simulink model "mg_simulator"  (Simulink 9.0)
settings: Solver=VariableStepAuto  StartTime=0.0  StopTime=Tsim  FixedStep=.005  MaxStep=Ts  RelTol=1e-6  EnableMultiTasking=on
InitFcn:
  | mg_simulator_init
values from neighbouring files (symbols this model uses):
  g_vector = [1 1 1 1]    [mg_simulator_init.m]
  Init = [305; 297; 315; 320]    [mg_simulator_init.m]
  N = 3    [mg_simulator_init.m]    (also in mpc_run_nodewise2.m = 6; mpc_run_nodewise3.m = 6; mpc_run_nodewise4.m = 6; mpc_run_nodewise_slow.m = 6)
  n_Q1 = .01    (= 0.01)    [mg_simulator_init.m]
  n_Q2 = n_Q1    (= 0.01)    [mg_simulator_init.m]
  n_Q3 = n_Q2    (= 0.01)    [mg_simulator_init.m]
  n_Q4 = n_Q3    (= 0.01)    [mg_simulator_init.m]
  Q = 10*eye    [mg_simulator_init.m]    (also in mpc_run_nodewise2.m; mpc_run_nodewise3.m; mpc_run_nodewise4.m; mpc_run_nodewise_slow.m)
  R = .1*eye    [mg_simulator_init.m]    (also in mpc_run_nodewise2.m = 0*eye; mpc_run_nodewise3.m = 0*eye; mpc_run_nodewise4.m = 0*eye; mpc_run_nodewise_slow.m = 0*eye)
  Thresh = 4    [mg_simulator_init.m]
  Ts = .01    (= 0.01)    [mg_simulator_init.m]    (also in mpc_run_nodewise2.m = 0.3; mpc_run_nodewise3.m = 0.3; mpc_run_nodewise4.m = 0.3; mpc_run_nodewise_slow.m = 0.3)
  v_ref = 310    [mg_simulator_init.m]    (also in mpc_run_nodewise2.m; mpc_run_nodewise3.m; mpc_run_nodewise4.m; mpc_run_nodewise_slow.m)
undefined symbols (not defined in the file or in its folder): mpc_run_nodewise_mdl_fast, mpc_run_nodewise_mdl_fast2, mpc_run_nodewise_mdl_fast3, mpc_run_nodewise_mdl_fast4, plecs
settings Model: SuppressorTable=22 serialization::archive 11 0 6 0 0 0 0 0  Creator=manaswini  LastModifiedBy=seananderson  ExtModeAutoUpdateStatusClock=off
settings DataIOCC: LimitDataPoints=on  SignalLoggingSaveFormat=ModelDataLogs
settings OptimizationCC: ExpressionDepthLimit=2147483647
settings DebuggingCC: AlgebraicLoopMsg=none  SaveWithParameterizedLinksMsg=none  MaxConsecutiveZCsMsg=none  SolverPrmCheckMsg=warning  FcnCallInpInsideContextMsg=warning  StateNameClashWarn=warning
settings HardwareCC: TargetHWDeviceType=32-bit Generic
settings GRTTargetCC: TargetFcnLib=ansi_tfl_tmw.mat  CombineOutputUpdateFcns=off  GRTInterface=on

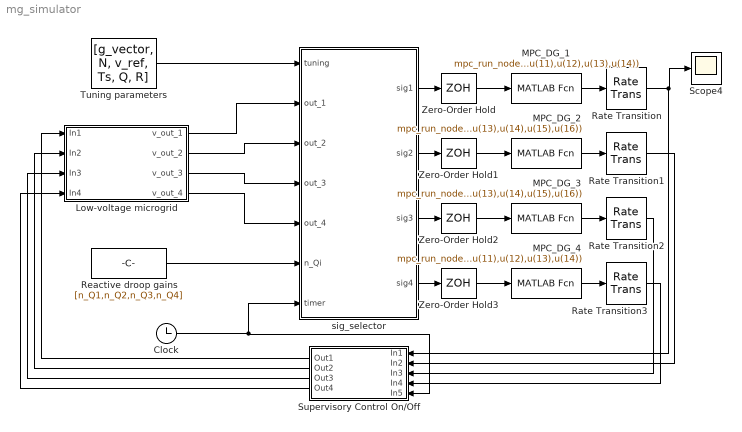
== system mg_simulator ==
  Clock : Clock
  Low-voltage microgrid : Subsystem  LoadFcn=plecs('sl', 200);  InitFcn=plecs('sl', 214);  StartFcn=plecs('sl', 208);  StopFcn=plecs('sl', 209);  mask(PlecsCircuit){PLECSData=<binary blob, 39660 chars, not shown>}
      mask prompts: PLECSData "PLECS Data (Do not delete or modify!)"
      mask init:
      | % PLACE CUSTOM INITIALIZATIONS ABOVE
      | % DO NOT REMOVE
      | plecs('sl', 215);
      | % DO NOT REMOVE
      settings: CopyFcn=plecs('sl', 203);  DeleteFcn=plecs('sl', 205);  UndoDeleteFcn=plecs('sl', 206);  PreSaveFcn=plecs('sl', 211);  PostSaveFcn=plecs('sl', 201);  NameChangeFcn=plecs('sl', 210);  DestroyFcn=plecs('sl', 207);  PreCopyFcn=plecs('sl', 216);  OpenFcn=plecs('sl', 202);  ErrorFcn=plerrorfcn
      mask Help: web(['file:///' fullfile(plecsdoc, 'creatingacircuit.html')])
      mask Display: disp('PLECS\nCircuit')
  MPC_DG_1 : MATLABFcn  MATLABFcn=mpc_run_nodewise_mdl_fast(u(1),u(2),u(3),u(4),u(5),u(6),u(7),u(8),u(9),u(10),u(11),u(12),u(13),u(14))  SampleTime=.02
  MPC_DG_2 : MATLABFcn  MATLABFcn=mpc_run_nodewise_mdl_fast2(u(1),u(2),u(3:4),u(5:6),u(7),u(8),u(9),u(10),u(11),u(12),u(13),u(14),u(15),u(16))  SampleTime=.02
  MPC_DG_3 : MATLABFcn  MATLABFcn=mpc_run_nodewise_mdl_fast3(u(1),u(2),u(3:4),u(5:6),u(7),u(8),u(9),u(10),u(11),u(12),u(13),u(14),u(15),u(16))  SampleTime=.02
  MPC_DG_4 : MATLABFcn  MATLABFcn=mpc_run_nodewise_mdl_fast4(u(1),u(2),u(3),u(4),u(5),u(6),u(7),u(8),u(9),u(10),u(11),u(12),u(13),u(14))  SampleTime=.02
  Rate Transition{,1..3} (4 alike) : RateTransition
  Reactive droop gains : Constant  Value=[n_Q1,n_Q2,n_Q3,n_Q4]
  Scope4 : Scope
  Supervisory Control On/Off : Subsystem
  Tuning parameters : Constant  Value=[g_vector, N, v_ref, Ts, Q, R]
  Zero-Order Hold{,1..3} (4 alike) : ZeroOrderHold  SampleTime=-1
  sig_selector : MATLAB Function  TreatAsAtomicUnit=on
  wires:
  Clock/1 -> sig_selector/7(timer), Supervisory Control On/Off/5(In5)
  Low-voltage microgrid/1(v_out_1) -> sig_selector/2(out_1)
  Low-voltage microgrid/2(v_out_2) -> sig_selector/3(out_2)
  Low-voltage microgrid/3(v_out_3) -> sig_selector/4(out_3)
  Tuning parameters/1 -> sig_selector/1(tuning)
  Low-voltage microgrid/4(v_out_4) -> sig_selector/5(out_4)
  Zero-Order Hold/1 -> MPC_DG_1/1
  sig_selector/1(sig1) -> Zero-Order Hold/1
  MPC_DG_1/1 -> Rate Transition/1
  Rate Transition/1 -> Supervisory Control On/Off/1(In1), Scope4/1
  Zero-Order Hold1/1 -> MPC_DG_2/1
  MPC_DG_2/1 -> Rate Transition1/1
  sig_selector/2(sig2) -> Zero-Order Hold1/1
  Zero-Order Hold2/1 -> MPC_DG_3/1
  MPC_DG_3/1 -> Rate Transition2/1
  sig_selector/3(sig3) -> Zero-Order Hold2/1
  Zero-Order Hold3/1 -> MPC_DG_4/1
  MPC_DG_4/1 -> Rate Transition3/1
  sig_selector/4(sig4) -> Zero-Order Hold3/1
  Rate Transition1/1 -> Supervisory Control On/Off/2(In2)
  Rate Transition2/1 -> Supervisory Control On/Off/3(In3)
  Rate Transition3/1 -> Supervisory Control On/Off/4(In4)
  Supervisory Control On/Off/1(Out1) -> Low-voltage microgrid/1(In1)
  Supervisory Control On/Off/2(Out2) -> Low-voltage microgrid/2(In2)
  Supervisory Control On/Off/3(Out3) -> Low-voltage microgrid/3(In3)
  Supervisory Control On/Off/4(Out4) -> Low-voltage microgrid/4(In4)
  Reactive droop gains/1 -> sig_selector/6(n_Qi)

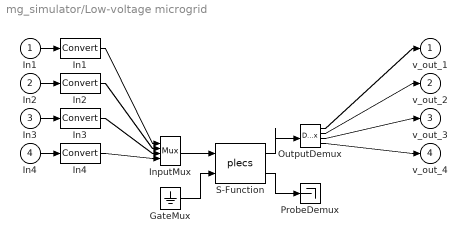
== system mg_simulator/Low-voltage microgrid ==
  In1 : Inport  PortDimensions=1
  In2 : Inport  Port=2  PortDimensions=1
  In3 : Inport  Port=3  PortDimensions=1
  In4 : Inport  Port=4  PortDimensions=1
  " GateMux " : Ground
  " In1 " : DataTypeConversion  SaturateOnIntegerOverflow=on  RndMeth=Zero
  " In2 " : DataTypeConversion  SaturateOnIntegerOverflow=on  RndMeth=Zero
  " In3 " : DataTypeConversion  SaturateOnIntegerOverflow=on  RndMeth=Zero
  " In4 " : DataTypeConversion  SaturateOnIntegerOverflow=on  RndMeth=Zero
  " InputMux " : Mux  Inputs=[ 1 1 1 1 ]
  " OutputDemux " : Demux  Outputs=[ 1 1 1 1 ]
  " ProbeDemux " : Terminator
  " S-Function " : S-Function  FunctionName=plecs  SFunctionDeploymentMode=off  EnableBusSupport=off
  v_out_1 : Outport  PortDimensions=1
  v_out_2 : Outport  Port=2  PortDimensions=1
  v_out_3 : Outport  Port=3  PortDimensions=1
  v_out_4 : Outport  Port=4  PortDimensions=1
  wires:
  " S-Function "/2 -> " ProbeDemux "/1
  " GateMux "/1 -> " S-Function "/2
  " InputMux "/1 -> " S-Function "/1
  " S-Function "/1 -> " OutputDemux "/1
  In1/1 -> " In1 "/1
  " In1 "/1 -> " InputMux "/1
  In2/1 -> " In2 "/1
  " In2 "/1 -> " InputMux "/2
  In3/1 -> " In3 "/1
  " In3 "/1 -> " InputMux "/3
  In4/1 -> " In4 "/1
  " In4 "/1 -> " InputMux "/4
  " OutputDemux "/1 -> v_out_1/1
  " OutputDemux "/2 -> v_out_2/1
  " OutputDemux "/3 -> v_out_3/1
  " OutputDemux "/4 -> v_out_4/1

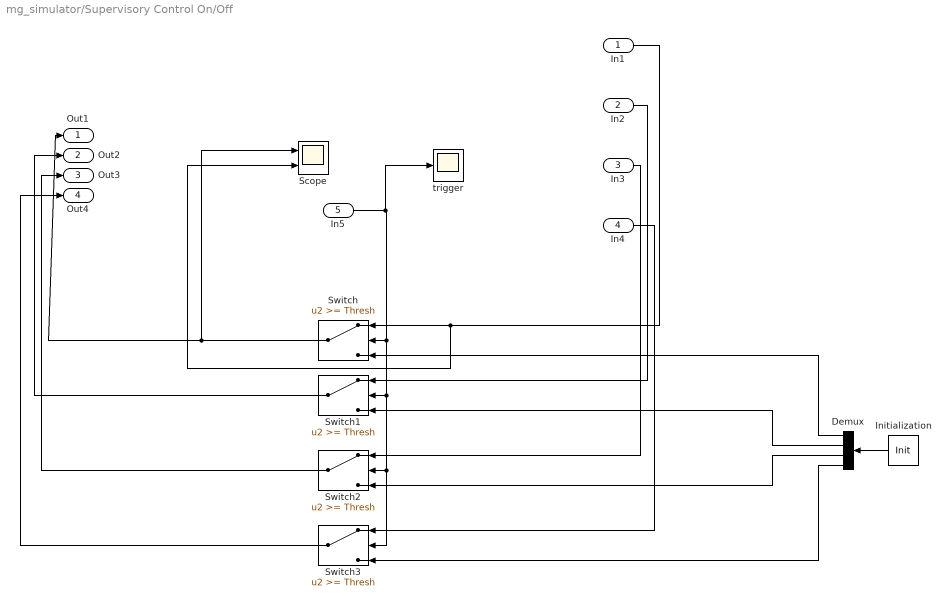
== system mg_simulator/Supervisory Control On/Off ==
  In1 : Inport
  In2 : Inport  Port=2
  In3 : Inport  Port=3
  In4 : Inport  Port=4
  In5 : Inport  Port=5
  Demux : Demux
  Initialization : Constant  Value=Init
  Scope : Scope  NumInputPorts=2
  Switch{,1..3} (4 alike) : Switch  Threshold=Thresh
  trigger : Scope
  Out1 : Outport
  Out2 : Outport  Port=2
  Out3 : Outport  Port=3
  Out4 : Outport  Port=4
  wires:
  Switch3/1 -> Out4/1
  In3/1 -> Switch2/1
  Demux/2 -> Switch1/3
  In4/1 -> Switch3/1
  Demux/1 -> Switch/3
  Initialization/1 -> Demux/1
  Demux/4 -> Switch3/3
  Switch2/1 -> Out3/1
  Switch/1 -> Scope/1, Out1/1
  In2/1 -> Switch1/1
  Demux/3 -> Switch2/3
  Switch1/1 -> Out2/1
  In5/1 -> trigger/1, Switch3/2, Switch2/2, Switch1/2, Switch/2
  In1/1 -> Scope/2, Switch/1

== matlab function sig_selector ==
  data: sig1 output double; tuning input double; out_1 input double; out_2 input double; out_3 input double; out_4 input double; n_Qi input double; sig2 output double; sig3 output double; sig4 output double; timer input double
function [sig1, sig2, sig3, sig4] = selector(tuning, out_1, out_2,...
                                            out_3, out_4, n_Qi, timer)
% tuning = [g_vector, N, v_ref, Ts, Q, R];
g = tuning(1:4);
N = tuning(5);
v_ref = tuning(6);
Ts = tuning(7);
Q = tuning(8);
R = tuning(9);
Q_L_i = 0;
Q_di = 0;

sig1 = [g(1), out_1, out_2, 2, 1, ...
    N, v_ref, n_Qi(1), Q_L_i, Q_di, Ts, Q, R, timer]';
sig2 = [g(2), out_2, [out_1 out_3], [1 3], 2, ...
    N, v_ref, n_Qi(2), Q_L_i, Q_di, Ts, Q, R, timer]';
sig3 = [g(3), out_3, [out_2 out_4], [2 4], 3, ...
    N, v_ref, n_Qi(3), Q_L_i, Q_di, Ts, Q, R, timer]';
sig4 = [g(4), out_4, out_3, 3, 4, ...
    N, v_ref, n_Qi(4), Q_L_i, Q_di, Ts, Q, R, timer]';

end
